simulink model "workshop_complete"  (R2018b)
settings: Solver=FixedStepAuto  StartTime=0.0  StopTime=Inf  RelTol=1e-3  EnableMultiTasking=on
libraries: arduinolib x5
settings Model: SimulationMode=external  ExtModeTrigDuration=2  Creator=Admin  LastModifiedBy=Admin
settings OptimizationCC: EnhancedBackFolding=on  PassReuseOutputArgsAs=Individual arguments  MaxStackSize=64  OptimizeBlockOrder=speed  DifferentSizesBufferReuse=on  OptimizationCustomize=off
settings DebuggingCC: ParameterTunabilityLossMsg=error
settings HardwareCC: ProdBitPerPointer=32  ProdBitPerSizeT=32  ProdBitPerPtrDiffT=32  ProdLargestAtomicInteger=Long  ProdLargestAtomicFloat=Double  ProdWordSize=32  ProdHWDeviceType=ARM Compatible->ARM Cortex
settings SFSimCC: MATLABDynamicMemAlloc=off
settings RTWCC: SystemTargetFile=ert.tlc  HardwareBoard=Arduino Due  TemplateMakefile=ert_default_tmf  GenerateReport=on  Toolchain=Arduino ARM  BuildConfiguration=Faster Runs  IncludeHyperlinkInReport=on  LaunchReport=on  GenerateTraceInfo=on  GenerateTraceReport=on  GenerateTraceReportSl=on  GenerateTraceReportSf=on  GenerateTraceReportEml=on
settings CodeAppCC: ForceParamTrailComments=on  IgnoreCustomStorageClasses=off  OperatorAnnotations=on  SimulinkDataObjDesc=on  SFDataObjDesc=on  InsertBlockDesc=on
settings ERTTargetCC: SupportContinuousTime=on  SupportVariableSizeSignals=on  ExtMode=on  ExtModeMexArgs='127.0.0.1' 0 17725

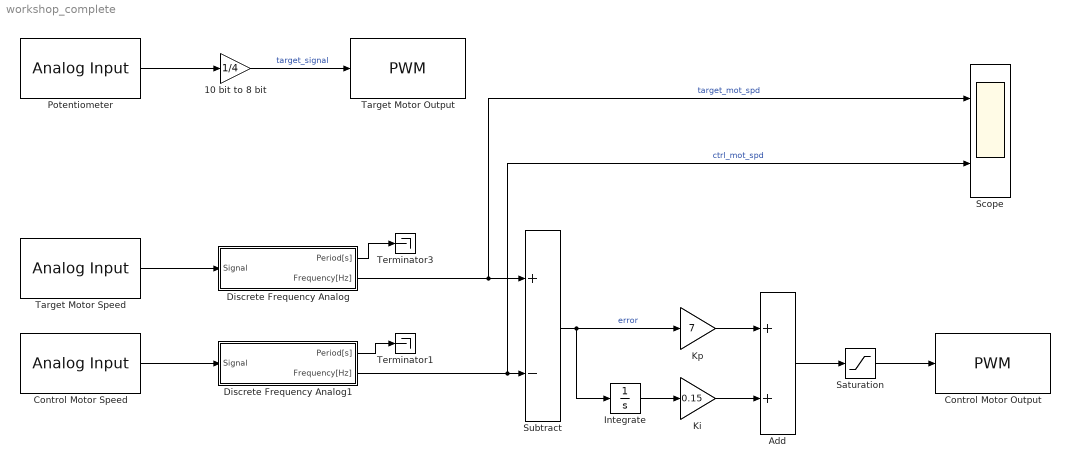
== system workshop_complete ==
  10 bit to 8 bit : Gain  Gain=1/4
  Add : Sum
  Control Motor Output : arduinolib/PWM  pinNumber=3  EnableInputFrequency=off  InitialFrequency=2000  InitialDutyCycle=0  NotificationType=None  blockPlatform=arduino
  Control Motor Speed : arduinolib/Analog Input  pinNumber=2  ReadResultsOnly=off  ConversionTriggerSource=Software  ExternalTriggerType=uint32(0)  OutputDataType=uint16  EnableConversionCompleteNotify=off  EnableOuputStatus=off  SampleTime=0.001  blockPlatform=arduino
  Discrete Frequency Analog : Subsystem  mask{sampleTime=0.001, threshold=700}
      mask prompts: sampleTime "Sample Time [s]"
  Discrete Frequency Analog1 : Subsystem  mask{sampleTime=0.001, threshold=700}
      mask prompts: sampleTime "Sample Time [s]"
  Integrate : Integrator
  Ki : Gain  Gain=0.15
  Kp : Gain  Gain=7
  Potentiometer : arduinolib/Analog Input  pinNumber=0  ReadResultsOnly=off  ConversionTriggerSource=Software  ExternalTriggerType=uint32(0)  OutputDataType=uint16  EnableConversionCompleteNotify=off  EnableOuputStatus=off  SampleTime=0.001  blockPlatform=arduino
  Saturation : Saturate  UpperLimit=255  LowerLimit=0
  Scope : Scope  NumInputPorts=2
  Subtract : Sum  Inputs=+-
  Target Motor Output : arduinolib/PWM  pinNumber=2  EnableInputFrequency=off  InitialFrequency=2000  InitialDutyCycle=0  NotificationType=None  blockPlatform=arduino
  Target Motor Speed : arduinolib/Analog Input  pinNumber=3  ReadResultsOnly=off  ConversionTriggerSource=Software  ExternalTriggerType=uint32(0)  OutputDataType=uint16  EnableConversionCompleteNotify=off  EnableOuputStatus=off  SampleTime=0.001  blockPlatform=arduino
  Terminator1 : Terminator
  Terminator3 : Terminator
  wires:
  Potentiometer/1 -> 10 bit to 8 bit/1
  Target Motor Speed/1 -> Discrete Frequency Analog/1(Signal)
  Control Motor Speed/1 -> Discrete Frequency Analog1/1(Signal)
  10 bit to 8 bit/1 -> Target Motor Output/1  "target_signal"
  Discrete Frequency Analog1/2(Frequency[Hz]) -> Scope/2, Subtract/2  "ctrl_mot_spd"
  Discrete Frequency Analog1/1(Period[s]) -> Terminator1/1
  Discrete Frequency Analog/2(Frequency[Hz]) -> Subtract/1, Scope/1  "target_mot_spd"
  Discrete Frequency Analog/1(Period[s]) -> Terminator3/1
  Subtract/1 -> Integrate/1, Kp/1  "error"
  Integrate/1 -> Ki/1
  Kp/1 -> Add/1
  Ki/1 -> Add/2
  Saturation/1 -> Control Motor Output/1
  Add/1 -> Saturation/1

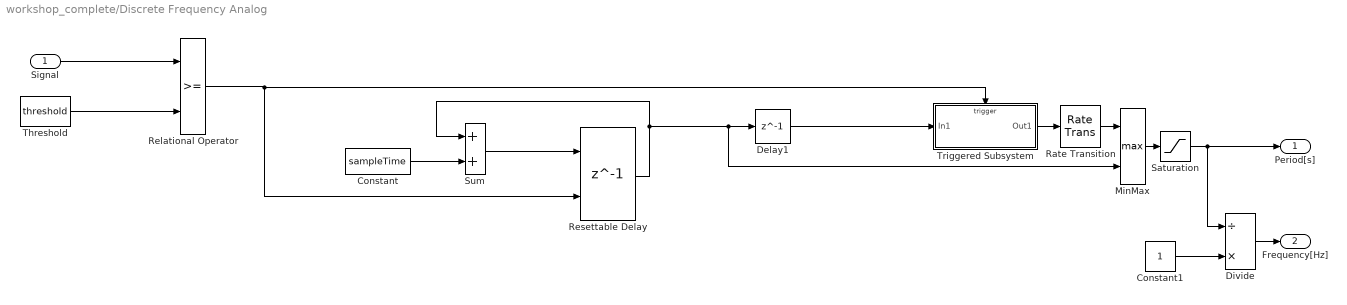
== system workshop_complete/Discrete Frequency Analog ==
  Signal : Inport
  Constant : Constant  Value=sampleTime
  Constant1 : Constant
  Delay1 : Delay  DelayLength=1
  Divide : Product  Inputs=/*
  MinMax : MinMax  Function=max  Inputs=2
  Rate Transition : RateTransition
  Relational Operator : RelationalOperator  OutDataTypeStr=boolean  RndMeth=Simplest
  Resettable Delay : Delay  DelayLength=1  InitialCondition=0  ExternalReset=Rising
      settings: InputPortMap=u0,r5
  Saturation : Saturate  UpperLimit=100  LowerLimit=0.001
  Sum : Sum
  Threshold : Constant  Value=threshold
  Triggered Subsystem : Subsystem  TreatAsAtomicUnit=on
  Period[s] : Outport
  Frequency[Hz] : Outport  Port=2
  wires:
  Divide/1 -> Frequency[Hz]/1
  Constant1/1 -> Divide/2
  Threshold/1 -> Relational Operator/2
  Resettable Delay/1 -> Sum/1, Delay1/1, MinMax/2
  Signal/1 -> Relational Operator/1
  Relational Operator/1 -> Triggered Subsystem/Trigger, Resettable Delay/2
  Sum/1 -> Resettable Delay/1
  Triggered Subsystem/1(Out1) -> Rate Transition/1
  Delay1/1 -> Triggered Subsystem/1(In1)
  Constant/1 -> Sum/2
  Rate Transition/1 -> MinMax/1
  Saturation/1 -> Period[s]/1, Divide/1
  MinMax/1 -> Saturation/1

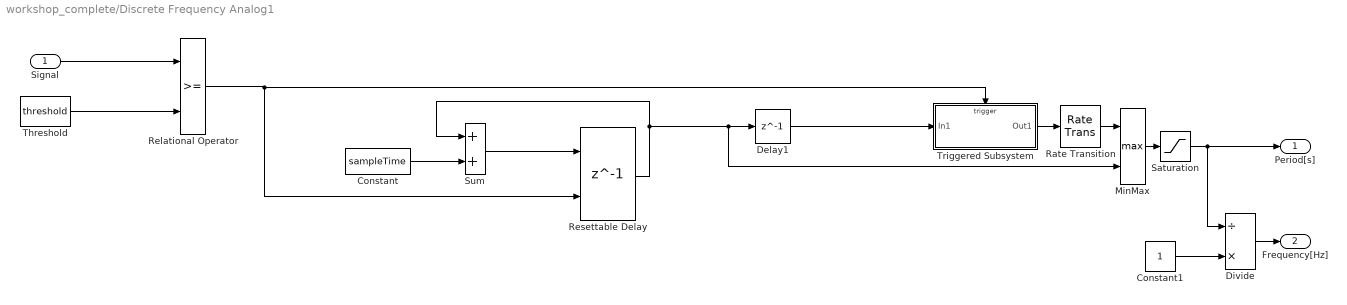
== system workshop_complete/Discrete Frequency Analog1 ==
  Signal : Inport
  Constant : Constant  Value=sampleTime
  Constant1 : Constant
  Delay1 : Delay  DelayLength=1
  Divide : Product  Inputs=/*
  MinMax : MinMax  Function=max  Inputs=2
  Rate Transition : RateTransition
  Relational Operator : RelationalOperator  OutDataTypeStr=boolean  RndMeth=Simplest
  Resettable Delay : Delay  DelayLength=1  InitialCondition=0  ExternalReset=Rising
      settings: InputPortMap=u0,r5
  Saturation : Saturate  UpperLimit=100  LowerLimit=0.001
  Sum : Sum
  Threshold : Constant  Value=threshold
  Triggered Subsystem : Subsystem  TreatAsAtomicUnit=on
  Period[s] : Outport
  Frequency[Hz] : Outport  Port=2
  wires:
  MinMax/1 -> Saturation/1
  Saturation/1 -> Divide/1, Period[s]/1
  Rate Transition/1 -> MinMax/1
  Constant/1 -> Sum/2
  Delay1/1 -> Triggered Subsystem/1(In1)
  Triggered Subsystem/1(Out1) -> Rate Transition/1
  Sum/1 -> Resettable Delay/1
  Relational Operator/1 -> Resettable Delay/2, Triggered Subsystem/Trigger
  Signal/1 -> Relational Operator/1
  Resettable Delay/1 -> MinMax/2, Delay1/1, Sum/1
  Threshold/1 -> Relational Operator/2
  Constant1/1 -> Divide/2
  Divide/1 -> Frequency[Hz]/1

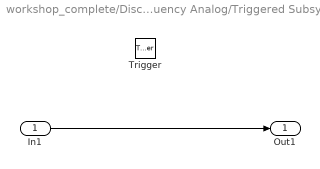
== system workshop_complete/Discrete Frequency Analog/Triggered Subsystem ==
  In1 : Inport
  Trigger : TriggerPort  VariantControl=Variant
  Out1 : Outport
  wires:
  In1/1 -> Out1/1

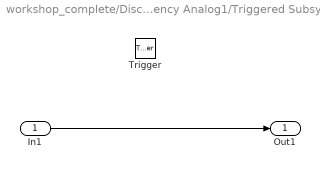
== system workshop_complete/Discrete Frequency Analog1/Triggered Subsystem ==
  In1 : Inport
  Trigger : TriggerPort  VariantControl=Variant
  Out1 : Outport
  wires:
  In1/1 -> Out1/1
